simulink model "untitled"  (R2022b)
settings: Solver=VariableStepAuto  StartTime=0.0  StopTime=500.0  RelTol=1e-3
settings Model: Creator=ADMIN  LastModifiedBy=ADMIN

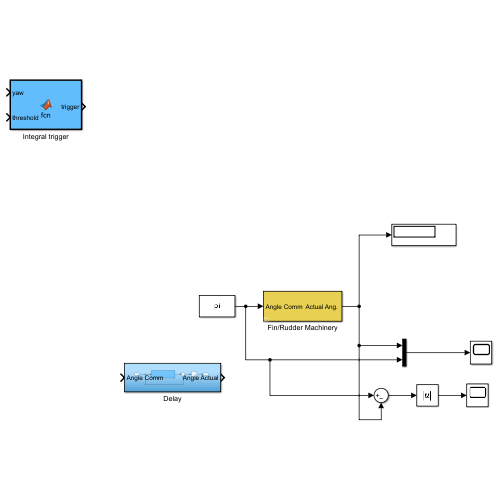
[thumbnail: Simulink's stored preview of the top-level diagram]
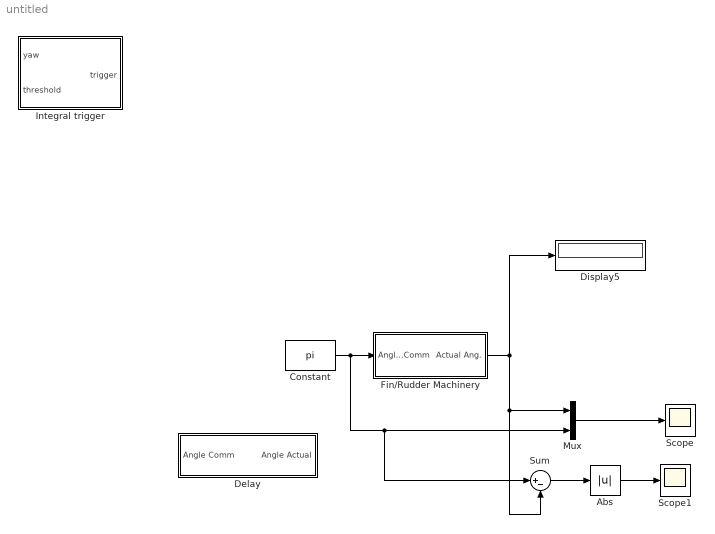
== system untitled ==
  Abs : Abs  SaturateOnIntegerOverflow=off
  Constant : Constant  Value=pi
  Delay : Subsystem
  Display5 : Display
  Fin/Rudder Machinery : Subsystem  AncestorBlock=mssSimulink/Modelling/Control Surfaces/Fin//Rudder Machinery  mask(Rudder Machinery){Dmax=pi, Dvmax=0.05, tc=.005}
      mask prompts: Dmax "Max. Rudder Angle (rad):"; Dvmax "Max. Rudder Rate (rad/sec.):"; tc "Time constant (sec):"
      mask help:
      | Model of van Amerongen for rudder machiery
      | Copyright (C) 2005 NTNU
      | Author: Tristan Perez
      settings: LibrarySourceBlock=mssSimulink/Modelling/Control Surfaces/Fin//Rudder Machinery
      mask Help: Rudder machinery model of Van Amerongen accounting for saturation and rate limit.
  Integral trigger : MATLAB Function  TreatAsAtomicUnit=on
  Mux : Mux  Inputs=2
  Scope : Scope
  Scope1 : Scope
  Sum : Sum  Inputs=|+-
  wires:
  Fin/Rudder Machinery/1("Actual Ang. ") -> Sum/2, Mux/1, Display5/1
  Constant/1 -> Sum/1, Mux/2, Fin/Rudder Machinery/1(Angle Comm)
  Mux/1 -> Scope/1
  Abs/1 -> Scope1/1
  Sum/1 -> Abs/1

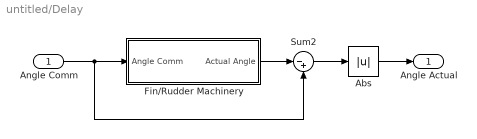
== system untitled/Delay ==
  Angle Comm : Inport
  Abs : Abs  SaturateOnIntegerOverflow=off
  Fin/Rudder Machinery : Subsystem  AncestorBlock=mssSimulink/Modelling/Control Surfaces/Fin//Rudder Machinery  mask(Rudder Machinery){Dmax=20, Dvmax=0.05, tc=.005}
      mask prompts: Dmax "Max. Rudder Angle (rad):"; Dvmax "Max. Rudder Rate (rad/sec.):"; tc "Time constant (sec):"
      mask help:
      | Model of van Amerongen for rudder machiery
      | Copyright (C) 2005 NTNU
      | Author: Tristan Perez
      settings: LibrarySourceBlock=mssSimulink/Modelling/Control Surfaces/Fin//Rudder Machinery
      mask Help: Rudder machinery model of Van Amerongen accounting for saturation and rate limit.
  Sum2 : Sum  Inputs=|-+
  Angle Actual : Outport
  wires:
  Sum2/1 -> Abs/1
  Angle Comm/1 -> Fin/Rudder Machinery/1(Angle Comm), Sum2/2
  Fin/Rudder Machinery/1("Actual Angle ") -> Sum2/1
  Abs/1 -> Angle Actual/1

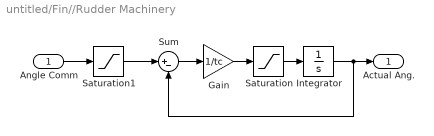
== system untitled/Fin//Rudder Machinery ==
  Angle Comm : Inport
  Gain : Gain  Gain=1/tc  SaturateOnIntegerOverflow=on  OutDataTypeStr=Inherit: Same as input  ParamDataTypeStr=Inherit: Same as input
  Integrator : Integrator
  Saturation : Saturate  UpperLimit=Dvmax  LowerLimit=-Dvmax
  Saturation1 : Saturate  UpperLimit=Dmax  LowerLimit=-Dmax
  Sum : Sum  Inputs=|+-  InputSameDT=on  SaturateOnIntegerOverflow=on  OutDataTypeStr=Inherit: Same as first input
  "Actual Ang. " : Outport  VectorParamsAs1DForOutWhenUnconnected=off
  wires:
  Gain/1 -> Saturation/1
  Sum/1 -> Gain/1
  Integrator/1 -> Sum/2, "Actual Ang. "/1
  Saturation1/1 -> Sum/1
  Saturation/1 -> Integrator/1
  Angle Comm/1 -> Saturation1/1

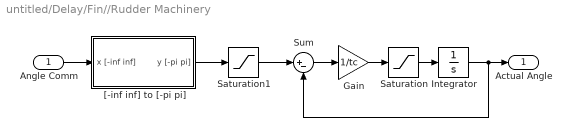
== system untitled/Delay/Fin//Rudder Machinery ==
  Angle Comm : Inport
  Gain : Gain  Gain=1/tc  SaturateOnIntegerOverflow=on  OutDataTypeStr=Inherit: Same as input  ParamDataTypeStr=Inherit: Same as input
  Integrator : Integrator
  Saturation : Saturate  UpperLimit=Dvmax  LowerLimit=-Dvmax
  Saturation1 : Saturate  UpperLimit=Dmax  LowerLimit=-Dmax
  Sum : Sum  Inputs=|+-  InputSameDT=on  SaturateOnIntegerOverflow=on  OutDataTypeStr=Inherit: Same as first input
  "[-inf inf] to [-pi pi]" : Subsystem  AncestorBlock=mssSimulink/Utilities/Math Operations/[-inf inf] to [-pi pi]  mask([-inf inf] to [-pi pi]){}
      mask help: Converts an angle in rad to (-pi pi)
      settings: LibrarySourceBlock=mssSimulink/Utilities/Math Operations/[-inf inf] to [-pi pi]
  "Actual Angle " : Outport  VectorParamsAs1DForOutWhenUnconnected=off
  wires:
  Gain/1 -> Saturation/1
  Sum/1 -> Gain/1
  Integrator/1 -> Sum/2, "Actual Angle "/1
  Saturation1/1 -> Sum/1
  Saturation/1 -> Integrator/1
  Angle Comm/1 -> "[-inf inf] to [-pi pi]"/1(x [-inf inf])
  "[-inf inf] to [-pi pi]"/1(y [-pi pi]) -> Saturation1/1

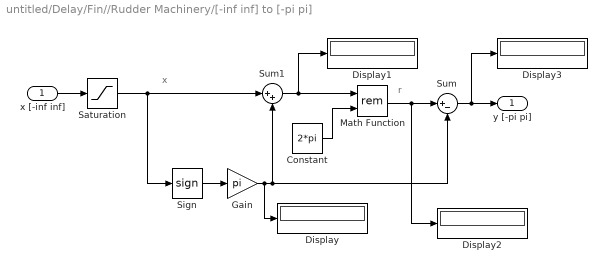
== system untitled/Delay/Fin//Rudder Machinery/[-inf inf] to [-pi pi] ==
  note: x
  note: r
  x [-inf inf] : Inport
  Constant : Constant  Value=2*pi
  Display{,1..3} (4 alike) : Display
  Gain : Gain  Gain=pi  SaturateOnIntegerOverflow=on  OutDataTypeStr=Inherit: Same as input  ParamDataTypeStr=Inherit: Same as input
  Math Function : Math  Operator=rem  SignedPower=on
  Saturation : Saturate  UpperLimit=1e10  LowerLimit=-1e10
  Sign : Signum
  Sum : Sum  Inputs=|+-  SaturateOnIntegerOverflow=on
  Sum1 : Sum  Inputs=|++  SaturateOnIntegerOverflow=on
  y [-pi pi] : Outport  VectorParamsAs1DForOutWhenUnconnected=off
  wires:
  x [-inf inf]/1 -> Saturation/1
  Sign/1 -> Gain/1
  Gain/1 -> Display/1, Sum/2, Sum1/2
  Sum1/1 -> Display1/1, Math Function/1
  Constant/1 -> Math Function/2
  Sum/1 -> Display3/1, y [-pi pi]/1
  Saturation/1 -> Sum1/1, Sign/1
  Math Function/1 -> Display2/1, Sum/1

== matlab function untitled/Integral trigger ==
  data: yaw input; trigger output; threshold input
function trigger = fcn(yaw, threshold)

if abs(yaw) < threshold
   trigger = 0;   % Trigger Integral part of PID
else
   trigger = 1;   % Stop Integral part of PID
end

end
